simulink model "unstable"  (Simulink 8.0)
settings: Solver=FixedStepDiscrete  StartTime=0.0  StopTime=Inf  FixedStep=.001  RelTol=1e-3
undefined symbols (not defined in the file or in its folder): dfilt
libraries: limblab x11, xpclib x5, xpcnilib x4, dsparch4 x4, dspsigops x2, simulink x2, xpcmeasurementcomputinglib x2, IntelSMIlibR2007b x1
CloseFcn:
  | rtwprivate ssgencode ModelCloseRequest rwalk_multi_local_v1
settings Model: Creator=limblab  LastModifiedBy=system administrator  ParamWorkspaceSource=ReferencedWorkspace  ExtModeArmWhenConnect=off  BufferReuse=off
settings DataIOCC: LimitDataPoints=off  SaveFormat=StructureWithTime  SignalLoggingSaveFormat=ModelDataLogs  SaveState=on  SignalLoggingName=sigsOut
settings OptimizationCC: BlockReduction=off  BooleanDataType=off  OptimizeBlockIOStorage=off  BufferReuse=off  ExpressionFolding=off  FoldNonRolledExpr=off  LocalBlockOutputs=off  InitFltsAndDblsToZero=on
settings DebuggingCC: SaveWithParameterizedLinksMsg=none  SignalResolutionControl=TryResolveAllWithWarning  SolverPrmCheckMsg=none  MultiTaskDSMMsg=warning  MultiTaskCondExecSysMsg=none  FcnCallInpInsideContextMsg=UseLocalSettings  StrictBusMsg=None
settings HardwareCC: ProdIntDivRoundTo=Zero  ProdEndianess=LittleEndian  ProdHWDeviceType=Generic->32-bit x86 compatible  TargetIntDivRoundTo=Floor  TargetEndianess=LittleEndian  TargetHWDeviceType=32-bit xPC Target (Intel Pentium)
settings SFSimCC: SimParseCustomCode=off
settings RTWCC: SystemTargetFile=xpctarget.tlc  TemplateMakefile=xpc_default_tmf  Description=xPC Target  GenerateReport=on  ProcessScript=xpctarget_make_rtw_hook  CustomSource=targets.c  IncludeERTFirstTime=on  RTWCompilerOptimization=On
settings xpcTargetCC: TargetFcnLib=ansi_tfl_tmw.mat  CodeReplacementLibrary=XPC_BLAS  ParMdlRefBuildCompliant=on  ConcurrentExecutionCompliant=on  CombineSignalStateStructs=off  GRTInterface=on  xPCTaskExecutionProfile=off  xPCRL32EventNumber=5000  xPCisDownloadable=off  xPCLoadParamSetFile=off  xPCConcurrentTasks=off  xPCEnableSFAnimation=off

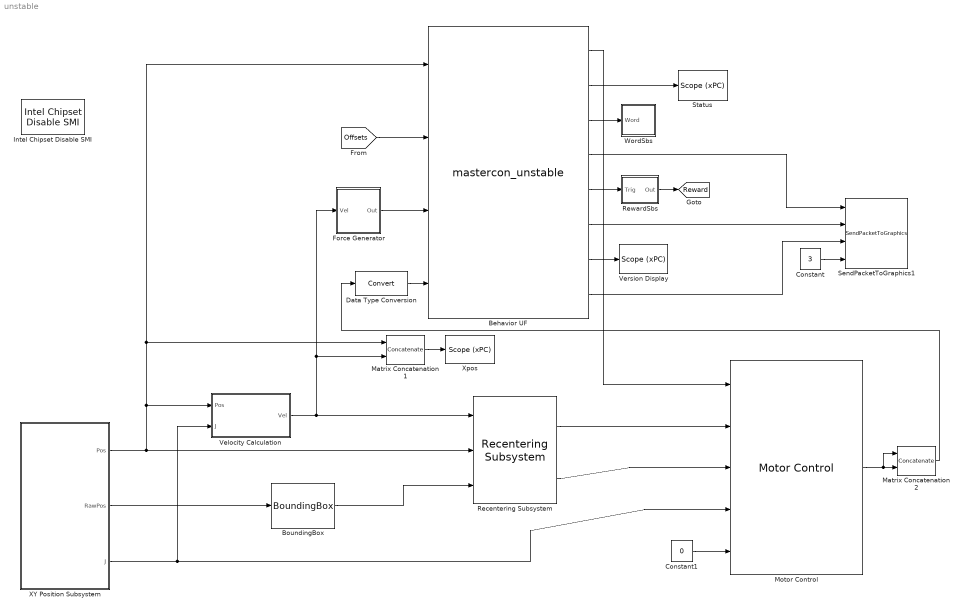
== system unstable ==
  Behavior UF : S-Function  FunctionName=mastercon_unstable  Parameters="0 1 1 2 1 1   5 10   0 0 0 0 0 0 0   .2 0 1 0   1 1  1   0 1 0 0  0.001   1 0   1 1.57   0   1 1   0 0   0"  EnableBusSupport=off
      mask Display:
      | disp('Master Control')
      | port_label('input',1,'pos')
      | port_label('input',2,'pos offsets')
      | port_label('input',3,'force')
      | port_label('input',4,'task off')
      | port_label('output',1,'force')
      | port_label('output',2,'status')
      | port_label('output',3,'word')
      | port_label('output',4,'targets')
      | port_label('output',5,'reward')
      | port_label('output',6,'tone')
      | port_label('output',7,'version')
      | port_label('output',8,'pos')
  BoundingBox : limblab/BoundingBox
  Constant : Constant  Value=3
  Constant1 : Constant  Value=0
  Data Type Conversion : DataTypeConversion
  Force Generator : Subsystem
  Intel Chipset Disable SMI : IntelSMIlibR2007b/Intel Chipset Disable SMI
  Matrix Concatenation1 : Concatenate
  Matrix Concatenation2 : Concatenate
  Motor Control : limblab/Motor Control
  Recentering Subsystem : limblab/Recentering Subsystem
  RewardSbs : Subsystem
  SendPacketToGraphics1 : limblab/SendPacketToGraphics
  Status : xpclib/Misc./Scope (xPC)   scopeno=3  scopetype=Target  autostart=on  viewmode=Numerical  formatstr='%6.0f state,%6.0f rewards,%6.0f aborts,%6.0f bump_ang,%6.0f debug_var'  grid=on  ylimits=[-10,10]  nosamples=10  noprepostsamples=0  interleave=10  triggermode=FreeRun  triggersignal=1  triggerlevel=0.0  triggerslope=Either  triggerscope=1  triggersample=0  filename=data.dat  mode=Lazy  writesize=512  autorestart=off  dynamicfilemode=off  maxwritefilesize=512*1024^2
  Velocity Calculation : Subsystem
  Version Display : xpclib/Misc./Scope (xPC)   scopeno=7  scopetype=Target  autostart=on  viewmode=Numerical  formatstr='%6.0f major,%6.0f minor,%6.0f revision,%6.0f build'  grid=on  ylimits=[-10,10]  nosamples=10  noprepostsamples=0  interleave=10  triggermode=FreeRun  triggersignal=1  triggerlevel=0.0  triggerslope=Either  triggerscope=1  triggersample=0  filename=data.dat  mode=Lazy  writesize=512  autorestart=off  dynamicfilemode=off  maxwritefilesize=512*1024^2
  WordSbs : Subsystem
  XY Position Subsystem : Subsystem
  Xpos : xpclib/Misc./Scope (xPC)   scopeno=1  scopetype=Target  autostart=on  viewmode=Numerical  formatstr='%15.2f X,%15.2f Y,%15.2f dX,%15.2f dY,%15.2f Fx,%15.2f Fy'  grid=on  ylimits=[-10,10]  nosamples=10  noprepostsamples=0  interleave=10  triggermode=FreeRun  triggersignal=1  triggerlevel=0.0  triggerslope=Either  triggerscope=1  triggersample=0  filename=data.dat  mode=Lazy  writesize=512  autorestart=off  dynamicfilemode=off  maxwritefilesize=512*1024^2
  tag scope: Reward=global
  wires:
  Velocity Calculation/1(Vel) -> Recentering Subsystem/1, Matrix Concatenation1/2, Force Generator/1(Vel)
  XY Position Subsystem/1(Pos) -> Recentering Subsystem/2, Velocity Calculation/1(Pos), Matrix Concatenation1/1, Behavior UF/1
  Behavior UF/2 -> Status/1
  Behavior UF/3 -> WordSbs/1(Word)
  Behavior UF/1 -> Motor Control/1
  Behavior UF/5 -> RewardSbs/1(Trig)
  BoundingBox/1 -> Recentering Subsystem/3
  XY Position Subsystem/3(J) -> Motor Control/4, Velocity Calculation/2(J)
  XY Position Subsystem/2(RawPos) -> BoundingBox/1
  Matrix Concatenation1/1 -> Xpos/1
  Recentering Subsystem/2 -> Motor Control/3
  Recentering Subsystem/1 -> Motor Control/2
  RewardSbs/1(Out) -> [Reward]
  Constant/1 -> SendPacketToGraphics1/4
  Behavior UF/4 -> SendPacketToGraphics1/1
  Force Generator/1(Out) -> Behavior UF/3
  [Offsets] -> Behavior UF/2
  Behavior UF/6 -> SendPacketToGraphics1/2
  Behavior UF/7 -> Version Display/1
  Behavior UF/8 -> SendPacketToGraphics1/3
  Motor Control/1 -> Matrix Concatenation2/1, Matrix Concatenation2/2
  Matrix Concatenation2/1 -> Data Type Conversion/1
  Data Type Conversion/1 -> Behavior UF/4
  Constant1/1 -> Motor Control/5

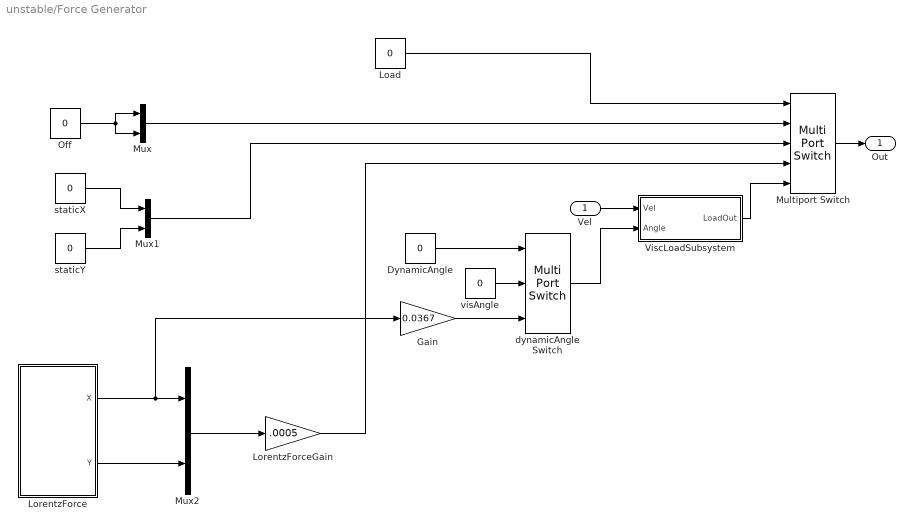
== system unstable/Force Generator ==
  Vel : Inport
  DynamicAngle : Constant  Value=0
  Gain : Gain  Gain=0.0367
  Load : Constant  Value=0
  LorentzForce : Subsystem
  LorentzForceGain : Gain  Gain=.0005
  Multiport Switch : MultiPortSwitch  DataPortOrder=Zero-based contiguous  Inputs=4  zeroidx=on
  Mux : Mux  Inputs=2
  Mux1 : Mux  Inputs=2
  Mux2 : Mux  Inputs=2
  Off : Constant  Value=0
  ViscLoadSubsystem : Subsystem
  dynamicAngle Switch : MultiPortSwitch  DataPortOrder=Zero-based contiguous  Inputs=2  zeroidx=on
  staticX : Constant  Value=0
  staticY : Constant  Value=0
  visAngle : Constant  Value=0
  Out : Outport
  wires:
  Off/1 -> Mux/2, Mux/1
  Multiport Switch/1 -> Out/1
  Mux/1 -> Multiport Switch/2
  Load/1 -> Multiport Switch/1
  Mux1/1 -> Multiport Switch/3
  staticX/1 -> Mux1/1
  staticY/1 -> Mux1/2
  LorentzForce/1(X) -> Mux2/1, Gain/1
  LorentzForce/2(Y) -> Mux2/2
  Mux2/1 -> LorentzForceGain/1
  LorentzForceGain/1 -> Multiport Switch/4
  Vel/1 -> ViscLoadSubsystem/1(Vel)
  ViscLoadSubsystem/1(LoadOut) -> Multiport Switch/5
  visAngle/1 -> dynamicAngle Switch/2
  DynamicAngle/1 -> dynamicAngle Switch/1
  dynamicAngle Switch/1 -> ViscLoadSubsystem/2(Angle)
  Gain/1 -> dynamicAngle Switch/3

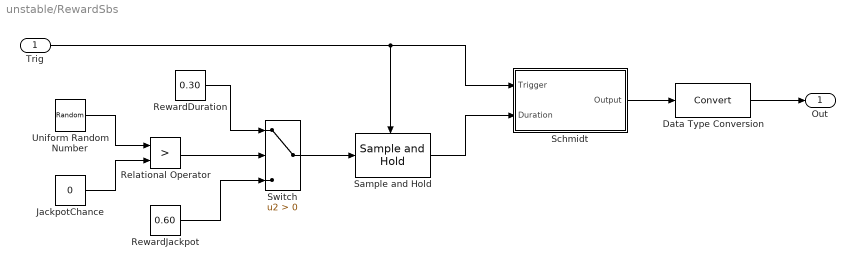
== system unstable/RewardSbs ==
  Trig : Inport
  Data Type Conversion : DataTypeConversion
  JackpotChance : Constant  Value=0
  Relational Operator : RelationalOperator  Operator=>  OutDataTypeStr=boolean
  RewardDuration : Constant  Value=0.30
  RewardJackpot : Constant  Value=0.60
  Sample and Hold : dspsigops/Sample and Hold  trig=Rising edge  initCond=0  latchinput=off
  Schmidt : Subsystem
  Switch : Switch  Criteria=u2 > Threshold  ZeroCross=off
  Uniform Random Number : UniformRandomNumber  Minimum=0  Maximum=100  SampleTime=0.001
  Out : Outport
  wires:
  Trig/1 -> Schmidt/1(Trigger), Sample and Hold/Trigger
  Data Type Conversion/1 -> Out/1
  Schmidt/1(Output) -> Data Type Conversion/1
  Sample and Hold/1 -> Schmidt/2(Duration)
  RewardJackpot/1 -> Switch/3
  Switch/1 -> Sample and Hold/1
  Uniform Random Number/1 -> Relational Operator/1
  Relational Operator/1 -> Switch/2
  JackpotChance/1 -> Relational Operator/2
  RewardDuration/1 -> Switch/1

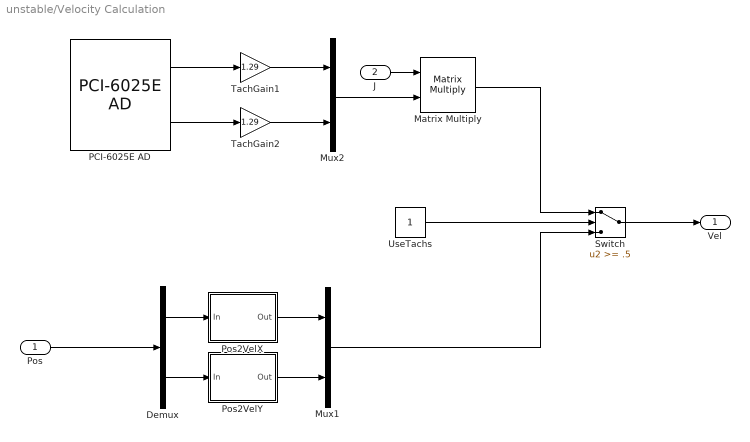
== system unstable/Velocity Calculation ==
  Pos : Inport
  J : Inport  Port=2
  Demux : Demux  Outputs=2
  Matrix Multiply : Product  Multiplication=Matrix(*)
  Mux1 : Mux  Inputs=2
  Mux2 : Mux  Inputs=2
  PCI-6025E AD : xpcnilib/A//D/E Series/PCI-6025E AD  channel=[1,2]  range=[-10,-10]  coupling=[0,0]  sampletime=0.001  slot=-1
  Pos2VelX : Subsystem
  Pos2VelY : Subsystem
  Switch : Switch  Threshold=.5
  TachGain1 : Gain  Gain=1.29
  TachGain2 : Gain  Gain=1.29
  UseTachs : Constant
  Vel : Outport
  wires:
  Pos2VelX/1(Out) -> Mux1/1
  Pos2VelY/1(Out) -> Mux1/2
  Demux/1 -> Pos2VelX/1(In)
  Demux/2 -> Pos2VelY/1(In)
  Pos/1 -> Demux/1
  UseTachs/1 -> Switch/2
  PCI-6025E AD/1 -> TachGain1/1
  PCI-6025E AD/2 -> TachGain2/1
  TachGain1/1 -> Mux2/1
  TachGain2/1 -> Mux2/2
  J/1 -> Matrix Multiply/1
  Mux2/1 -> Matrix Multiply/2
  Switch/1 -> Vel/1
  Mux1/1 -> Switch/3
  Matrix Multiply/1 -> Switch/1

== system unstable/WordSbs ==
  Word : Inport
  tag scope: Word=global
  wires:
  Word/1 -> [Word]

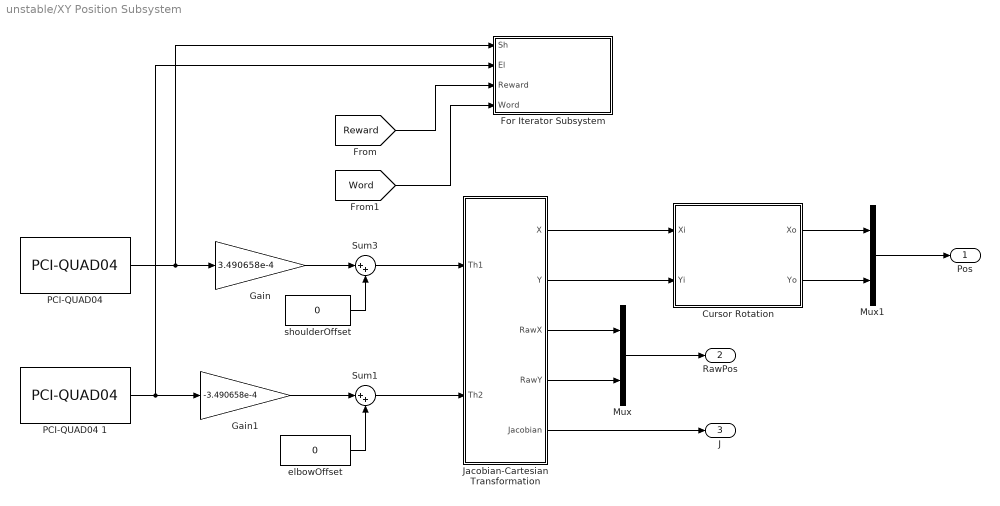
== system unstable/XY Position Subsystem ==
  Cursor Rotation : Subsystem
  For Iterator Subsystem : Subsystem  TreatAsAtomicUnit=on
  Gain : Gain  Gain=3.490658e-4
  Gain1 : Gain  Gain=-3.490658e-4
  Jacobian-Cartesian Transformation : Subsystem
  Mux : Mux  Inputs=2
  Mux1 : Mux  Inputs=2
  "PCI-QUAD04 " : xpcmeasurementcomputinglib/Incremental Encoder/PCI-QUAD04   channel=1  resetmode=on  polarity=Positive Index  mode=Normal  limit=0  range=-2^23...+2^23-1  speed=1x  prescale=0  ts=0.001  convbaseaddr=-1
  PCI-QUAD04 1 : xpcmeasurementcomputinglib/Incremental Encoder/PCI-QUAD04   channel=2  resetmode=on  polarity=Positive Index  mode=Normal  limit=0  range=-2^23...+2^23-1  speed=1x  prescale=0  ts=0.001  convbaseaddr=-1
  Sum1 : Sum  Inputs=|++  SaturateOnIntegerOverflow=on  InputSameDT=on  OutDataTypeStr=Inherit: Same as first input
  Sum3 : Sum  Inputs=|++  SaturateOnIntegerOverflow=on  InputSameDT=on  OutDataTypeStr=Inherit: Same as first input
  elbowOffset : Constant  Value=0
  shoulderOffset : Constant  Value=0
  Pos : Outport
  RawPos : Outport  Port=2
  J : Outport  Port=3
  wires:
  PCI-QUAD04 1/1 -> For Iterator Subsystem/2("El "), Gain1/1
  "PCI-QUAD04 "/1 -> For Iterator Subsystem/1(Sh), Gain/1
  Gain/1 -> Sum3/1
  Sum3/1 -> Jacobian-Cartesian Transformation/1(Th1)
  shoulderOffset/1 -> Sum3/2
  Gain1/1 -> Sum1/1
  elbowOffset/1 -> Sum1/2
  Sum1/1 -> Jacobian-Cartesian Transformation/2(Th2)
  Jacobian-Cartesian Transformation/1(X) -> Cursor Rotation/1(Xi)
  Jacobian-Cartesian Transformation/2(Y) -> Cursor Rotation/2(Yi)
  Cursor Rotation/1(Xo) -> Mux1/1
  Cursor Rotation/2(Yo) -> Mux1/2
  Jacobian-Cartesian Transformation/3(RawX) -> Mux/1
  Jacobian-Cartesian Transformation/4(RawY) -> Mux/2
  [Reward] -> For Iterator Subsystem/3(Reward)
  Jacobian-Cartesian Transformation/5(Jacobian) -> J/1
  Mux/1 -> RawPos/1
  Mux1/1 -> Pos/1
  [Word] -> For Iterator Subsystem/4(Word)

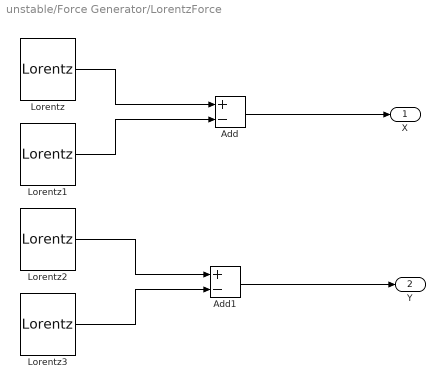
== system unstable/Force Generator/LorentzForce ==
  Add : Sum  Inputs=+-
  Add1 : Sum  Inputs=+-
  Lorentz : limblab/Lorentz  y0=.1
  Lorentz1 : limblab/Lorentz  y0=.2
  Lorentz2 : limblab/Lorentz  y0=.3
  Lorentz3 : limblab/Lorentz  y0=.4
  X : Outport
  Y : Outport  Port=2
  wires:
  Lorentz/1 -> Add/1
  Lorentz1/1 -> Add/2
  Add/1 -> X/1
  Lorentz2/1 -> Add1/1
  Lorentz3/1 -> Add1/2
  Add1/1 -> Y/1

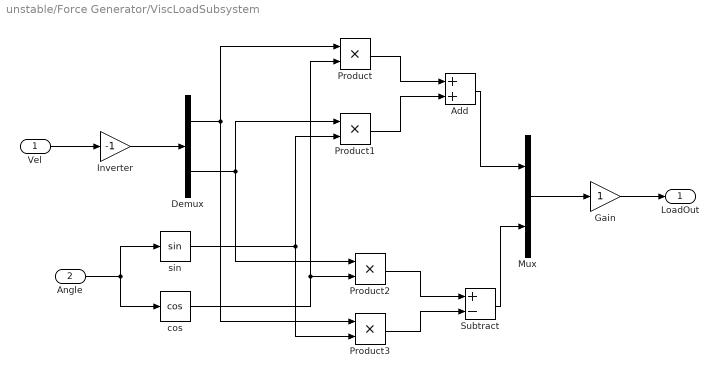
== system unstable/Force Generator/ViscLoadSubsystem ==
  Vel : Inport
  Angle : Inport  Port=2
  Add : Sum
  Demux : Demux  Outputs=2
  Gain : Gain
  Inverter : Gain  Gain=-1
  Mux : Mux  Inputs=2
  Product{,1..3} (4 alike) : Product  RndMeth=Zero
  Subtract : Sum  Inputs=+-
  cos : Trigonometry  Operator=cos
  sin : Trigonometry
  LoadOut : Outport
  wires:
  Mux/1 -> Gain/1
  Angle/1 -> sin/1, cos/1
  Add/1 -> Mux/1
  Subtract/1 -> Mux/2
  Product/1 -> Add/1
  Product1/1 -> Add/2
  Product2/1 -> Subtract/1
  Product3/1 -> Subtract/2
  Demux/1 -> Product/1, Product3/1
  cos/1 -> Product/2, Product2/2
  Demux/2 -> Product1/1, Product2/1
  sin/1 -> Product1/2, Product3/2
  Gain/1 -> LoadOut/1
  Vel/1 -> Inverter/1
  Inverter/1 -> Demux/1

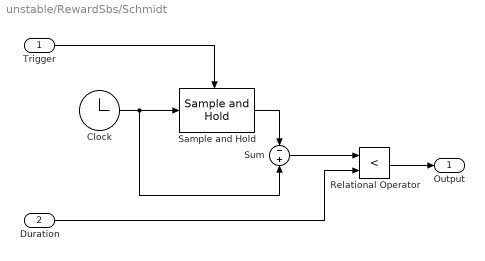
== system unstable/RewardSbs/Schmidt ==
  Trigger : Inport
  Duration : Inport  Port=2
  Clock : Clock
  Relational Operator : RelationalOperator  Operator=<  OutDataTypeStr=boolean
  Sample and Hold : dspsigops/Sample and Hold  trig=Rising edge  initCond=-1000  latchinput=off
  Sum : Sum  Inputs=-+
  Output : Outport
  wires:
  Clock/1 -> Sum/2, Sample and Hold/1
  Sample and Hold/1 -> Sum/1
  Sum/1 -> Relational Operator/1
  Duration/1 -> Relational Operator/2
  Relational Operator/1 -> Output/1
  Trigger/1 -> Sample and Hold/Trigger

== system unstable/Velocity Calculation/Pos2VelX ==
  In : Inport
  Derivative : Derivative
  Digital Filter : dsparch4/Digital Filter  TypePopup=FIR (all zeros)  IIRFiltStruct=Direct form II transposed  AllPoleFiltStruct=Direct form  FIRFiltStruct=Direct form  CoeffSource=Specify via dialog  NumCoeffs="[0.0144    0.0304    0.0724    0.1245    0.1668    0.1830    0.1668    0.1245    0.0724    0.0304    0.0144]"  DenCoeffs=[1 0.1]  BiQuadCoeffs=[1 0.3 0.4 1 0.1 0.2]  LatticeCoeffs=[0.2 0.4]  denIgnore=on  FiltPerSampPopup=One filter per frame  IC=0  ICnum=0  ICden=0  roundingMode=Floor  overflowMode=off  ScaleValues=1  scaleValueFracLength=14  stageInFracLength=15  stageOutFracLength=15  FilterSource=Specify via dialog  dfiltObjectName=dfilt.dffir([1 2 1])  InputProcessing=Inherited (this choice will be removed - see release notes)
  Digital Filter2 : dsparch4/Digital Filter  TypePopup=FIR (all zeros)  IIRFiltStruct=Direct form II transposed  AllPoleFiltStruct=Direct form  FIRFiltStruct=Direct form  CoeffSource=Specify via dialog  NumCoeffs="[0.0144    0.0304    0.0724    0.1245    0.1668    0.1830    0.1668    0.1245    0.0724    0.0304    0.0144]"  DenCoeffs=[1 0.1]  BiQuadCoeffs=[1 0.3 0.4 1 0.1 0.2]  LatticeCoeffs=[0.2 0.4]  denIgnore=on  FiltPerSampPopup=One filter per frame  IC=0  ICnum=0  ICden=0  roundingMode=Floor  overflowMode=off  ScaleValues=1  scaleValueFracLength=14  stageInFracLength=15  stageOutFracLength=15  FilterSource=Specify via dialog  dfiltObjectName=dfilt.dffir([1 2 1])  InputProcessing=Inherited (this choice will be removed - see release notes)
  dG : Gain  SampleTime=.001
  Out : Outport
  wires:
  Derivative/1 -> dG/1
  dG/1 -> Digital Filter/1
  Digital Filter2/1 -> Derivative/1
  In/1 -> Digital Filter2/1
  Digital Filter/1 -> Out/1

== system unstable/Velocity Calculation/Pos2VelY ==
  In : Inport
  Derivative : Derivative
  Digital Filter : dsparch4/Digital Filter  TypePopup=FIR (all zeros)  IIRFiltStruct=Direct form II transposed  AllPoleFiltStruct=Direct form  FIRFiltStruct=Direct form  CoeffSource=Specify via dialog  NumCoeffs="[0.0144    0.0304    0.0724    0.1245    0.1668    0.1830    0.1668    0.1245    0.0724    0.0304    0.0144]"  DenCoeffs=[1 0.1]  BiQuadCoeffs=[1 0.3 0.4 1 0.1 0.2]  LatticeCoeffs=[0.2 0.4]  denIgnore=on  FiltPerSampPopup=One filter per frame  IC=0  ICnum=0  ICden=0  roundingMode=Floor  overflowMode=off  ScaleValues=1  scaleValueFracLength=14  stageInFracLength=15  stageOutFracLength=15  FilterSource=Specify via dialog  dfiltObjectName=dfilt.dffir([1 2 1])  InputProcessing=Inherited (this choice will be removed - see release notes)
  Digital Filter2 : dsparch4/Digital Filter  TypePopup=FIR (all zeros)  IIRFiltStruct=Direct form II transposed  AllPoleFiltStruct=Direct form  FIRFiltStruct=Direct form  CoeffSource=Specify via dialog  NumCoeffs="[0.0144    0.0304    0.0724    0.1245    0.1668    0.1830    0.1668    0.1245    0.0724    0.0304    0.0144]"  DenCoeffs=[1 0.1]  BiQuadCoeffs=[1 0.3 0.4 1 0.1 0.2]  LatticeCoeffs=[0.2 0.4]  denIgnore=on  FiltPerSampPopup=One filter per frame  IC=0  ICnum=0  ICden=0  roundingMode=Floor  overflowMode=off  ScaleValues=1  scaleValueFracLength=14  stageInFracLength=15  stageOutFracLength=15  FilterSource=Specify via dialog  dfiltObjectName=dfilt.dffir([1 2 1])  InputProcessing=Inherited (this choice will be removed - see release notes)
  dG : Gain  SampleTime=.001
  Out : Outport
  wires:
  Derivative/1 -> dG/1
  dG/1 -> Digital Filter/1
  Digital Filter2/1 -> Derivative/1
  In/1 -> Digital Filter2/1
  Digital Filter/1 -> Out/1

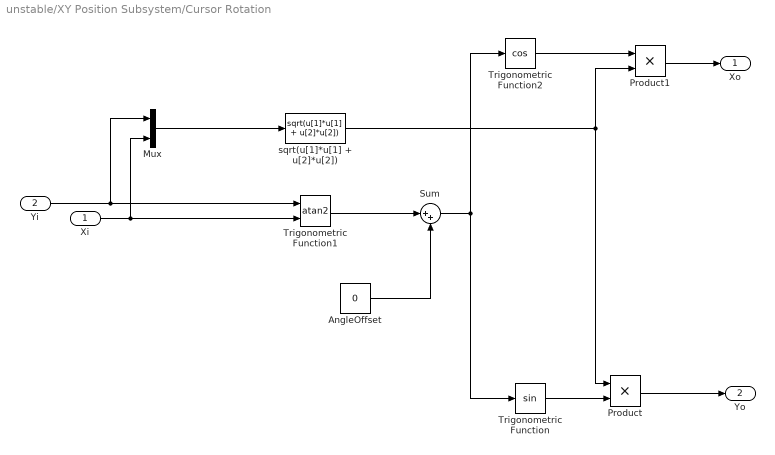
== system unstable/XY Position Subsystem/Cursor Rotation ==
  Xi : Inport
  Yi : Inport  Port=2
  AngleOffset : Constant  Value=0  SampleTime=.001
  Mux : Mux  Inputs=2
  Product : Product  RndMeth=Zero
  Product1 : Product  RndMeth=Zero
  Sum : Sum  Inputs=|++
  Trigonometric Function : Trigonometry
  Trigonometric Function1 : Trigonometry  Operator=atan2
  Trigonometric Function2 : Trigonometry  Operator=cos
  sqrt(u[1]*u[1] + u[2]*u[2]) : Fcn  Expr=sqrt(u[1]*u[1] + u[2]*u[2])
  Xo : Outport
  Yo : Outport  Port=2
  wires:
  AngleOffset/1 -> Sum/2
  Trigonometric Function1/1 -> Sum/1
  Yi/1 -> Trigonometric Function1/1, Mux/1
  Xi/1 -> Trigonometric Function1/2, Mux/2
  Mux/1 -> sqrt(u[1]*u[1] + u[2]*u[2])/1
  Trigonometric Function/1 -> Product/2
  Product/1 -> Yo/1
  sqrt(u[1]*u[1] + u[2]*u[2])/1 -> Product/1, Product1/2
  Sum/1 -> Trigonometric Function/1, Trigonometric Function2/1
  Product1/1 -> Xo/1
  Trigonometric Function2/1 -> Product1/1

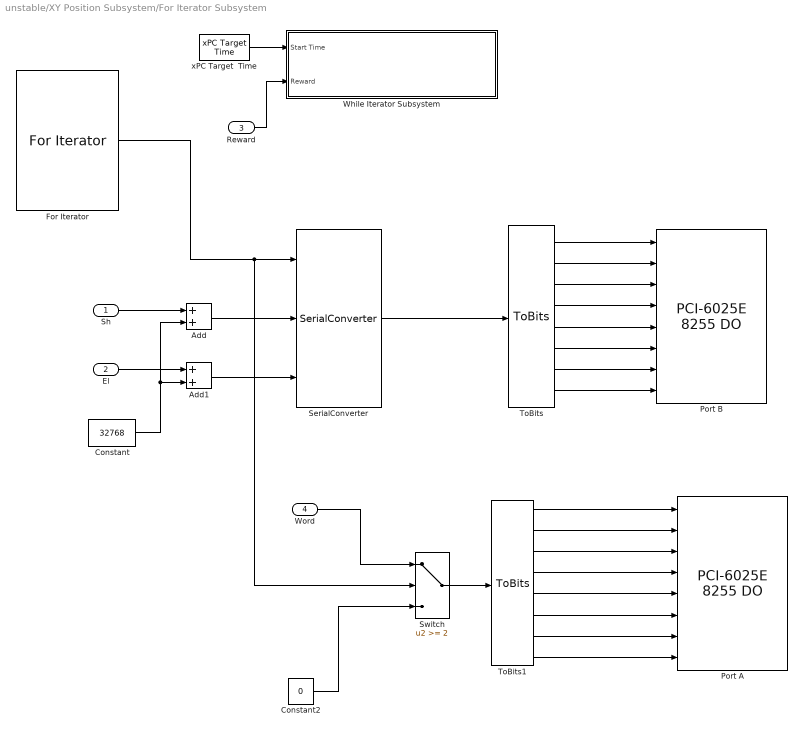
== system unstable/XY Position Subsystem/For Iterator Subsystem ==
  Sh : Inport
  "El " : Inport  Port=2
  Reward : Inport  Port=3
  Word : Inport  Port=4
  Add : Sum
  Add1 : Sum
  Constant : Constant  Value=32768
  Constant2 : Constant  Value=0
  For Iterator : ForIterator  IterationLimit=4  IndexMode=Zero-based  IterationVariableDataType=double
  Port A : xpcnilib/Digital Output/E Series/PCI-6025E 8255 DO  channel=1:8  port=A  reset=[1]  initValue=[0]  chip=1  sampletime=-1  slot=-1
  Port B : xpcnilib/Digital Output/E Series/PCI-6025E 8255 DO  channel=1:8  port=B  reset=[1]  initValue=[0]  chip=1  sampletime=-1  slot=-1
  SerialConverter : limblab/SerialConverter
  Switch : Switch  Threshold=2
  ToBits : limblab/ToBits
  ToBits1 : limblab/ToBits
  While Iterator Subsystem : Subsystem  TreatAsAtomicUnit=on
  "xPC Target  Time " : xpclib/Misc./xPC Target  Time   ts=-1
  wires:
  "xPC Target  Time "/1 -> While Iterator Subsystem/1(Start Time)
  SerialConverter/1 -> ToBits/1
  For Iterator/1 -> SerialConverter/1, Switch/2
  Sh/1 -> Add/1
  Add/1 -> SerialConverter/2
  Add1/1 -> SerialConverter/3
  "El "/1 -> Add1/1
  Constant/1 -> Add/2, Add1/2
  ToBits/1 -> Port B/1
  ToBits/2 -> Port B/2
  ToBits/3 -> Port B/3
  ToBits/4 -> Port B/4
  ToBits/5 -> Port B/5
  ToBits/6 -> Port B/6
  ToBits/7 -> Port B/7
  ToBits/8 -> Port B/8
  Reward/1 -> While Iterator Subsystem/2(Reward)
  ToBits1/1 -> Port A/1
  ToBits1/2 -> Port A/2
  ToBits1/3 -> Port A/3
  ToBits1/4 -> Port A/4
  ToBits1/5 -> Port A/5
  ToBits1/6 -> Port A/6
  ToBits1/7 -> Port A/7
  ToBits1/8 -> Port A/8
  Constant2/1 -> Switch/3
  Word/1 -> Switch/1
  Switch/1 -> ToBits1/1

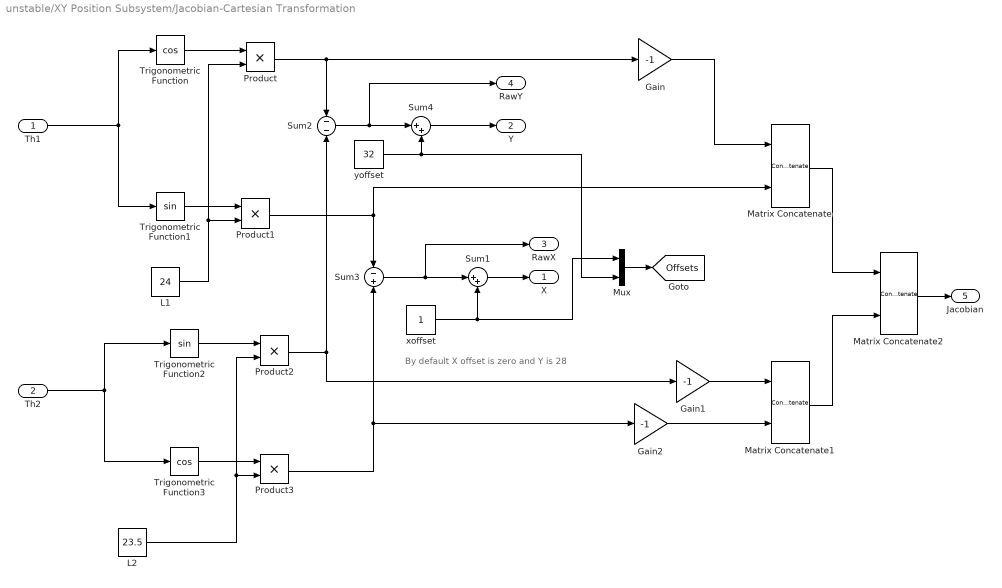
== system unstable/XY Position Subsystem/Jacobian-Cartesian Transformation ==
  note: By default X offset is zero and Y is 28
  Th1 : Inport
  Th2 : Inport  Port=2
  Gain : Gain  Gain=-1
  Gain1 : Gain  Gain=-1
  Gain2 : Gain  Gain=-1
  L1 : Constant  Value=24
  L2 : Constant  Value=23.5
  Matrix Concatenate : Concatenate  ConcatenateDimension=2
  Matrix Concatenate1 : Concatenate  ConcatenateDimension=2
  Matrix Concatenate2 : Concatenate  Mode=Multidimensional array  ConcatenateDimension=2
  Mux : Mux  Inputs=2
  Product{,1..3} (4 alike) : Product  RndMeth=Zero
  Sum1 : Sum  Inputs=|++  SaturateOnIntegerOverflow=on  InputSameDT=on  OutDataTypeStr=Inherit: Same as first input
  Sum2 : Sum  Inputs=--  SaturateOnIntegerOverflow=on  InputSameDT=on  OutDataTypeStr=Inherit: Same as first input
  Sum3 : Sum  Inputs=-+  SaturateOnIntegerOverflow=on  InputSameDT=on  OutDataTypeStr=Inherit: Same as first input
  Sum4 : Sum  Inputs=|++  SaturateOnIntegerOverflow=on  InputSameDT=on  OutDataTypeStr=Inherit: Same as first input
  Trigonometric Function : Trigonometry  Operator=cos
  Trigonometric Function1 : Trigonometry
  Trigonometric Function2 : Trigonometry
  Trigonometric Function3 : Trigonometry  Operator=cos
  xoffset : Constant
  yoffset : Constant  Value=32
  X : Outport
  Y : Outport  Port=2
  RawX : Outport  Port=3
  RawY : Outport  Port=4
  Jacobian : Outport  Port=5
  tag scope: Offsets=global
  wires:
  Th1/1 -> Trigonometric Function1/1, Trigonometric Function/1
  Product/1 -> Sum2/1, Gain/1
  Product2/1 -> Sum2/2, Gain1/1
  Sum3/1 -> Sum1/1, RawX/1
  Product1/1 -> Sum3/1, Matrix Concatenate/2
  Sum2/1 -> Sum4/1, RawY/1
  Sum4/1 -> Y/1
  Sum1/1 -> X/1
  xoffset/1 -> Sum1/2, Mux/1
  yoffset/1 -> Sum4/2, Mux/2
  Product3/1 -> Sum3/2, Gain2/1
  Th2/1 -> Trigonometric Function2/1, Trigonometric Function3/1
  Matrix Concatenate/1 -> Matrix Concatenate2/1
  Matrix Concatenate1/1 -> Matrix Concatenate2/2
  Matrix Concatenate2/1 -> Jacobian/1
  Gain/1 -> Matrix Concatenate/1
  Gain1/1 -> Matrix Concatenate1/1
  Gain2/1 -> Matrix Concatenate1/2
  Trigonometric Function/1 -> Product/1
  Trigonometric Function3/1 -> Product3/1
  Trigonometric Function2/1 -> Product2/1
  L2/1 -> Product2/2, Product3/2
  Trigonometric Function1/1 -> Product1/1
  L1/1 -> Product/2, Product1/2
  Mux/1 -> [Offsets]

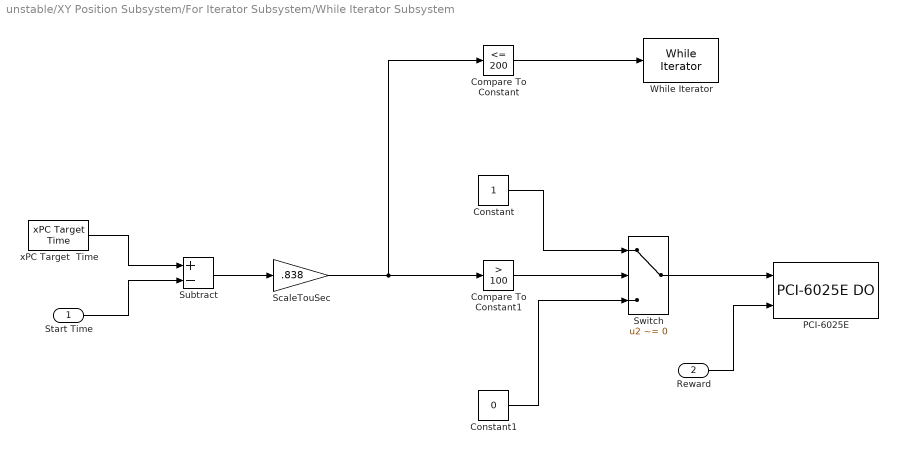
== system unstable/XY Position Subsystem/For Iterator Subsystem/While Iterator Subsystem ==
  Start Time : Inport
  Reward : Inport  Port=2
  Compare To Constant : simulink/Logic and Bit Operations/Compare To Constant  relop=<=  const=200  OutDataTypeStr=boolean
  Compare To Constant1 : simulink/Logic and Bit Operations/Compare To Constant  relop=>  const=100  OutDataTypeStr=boolean  ZeroCross=off
  Constant : Constant
  Constant1 : Constant  Value=0
  "PCI-6025E " : xpcnilib/Digital Output/E Series/PCI-6025E DO  channel=[1 2]  reset=[1]  initValue=[0]  sampletime=-1  slot=-1
  ScaleTouSec : Gain  Gain=.838
  Subtract : Sum  Inputs=+-
  Switch : Switch  Criteria=u2 ~= 0
  While Iterator : WhileIterator  MaxIters=-1  WhileBlockType=do-while
  "xPC Target  Time " : xpclib/Misc./xPC Target  Time   ts=-1
  wires:
  "xPC Target  Time "/1 -> Subtract/1
  Start Time/1 -> Subtract/2
  Subtract/1 -> ScaleTouSec/1
  Compare To Constant/1 -> While Iterator/1
  ScaleTouSec/1 -> Compare To Constant/1, Compare To Constant1/1
  Compare To Constant1/1 -> Switch/2
  Constant/1 -> Switch/1
  Constant1/1 -> Switch/3
  Switch/1 -> "PCI-6025E "/1
  Reward/1 -> "PCI-6025E "/2
